simulink model "ForcedPendulum"  (R2023a)
settings: Solver=VariableStepAuto  StartTime=0.0  StopTime=10.0  RelTol=1e-3
model workspace (MAT data in the model file):
  g = 9.8
  l = 0.5
settings Model: Creator=MY PC  LastModifiedBy=MY PC

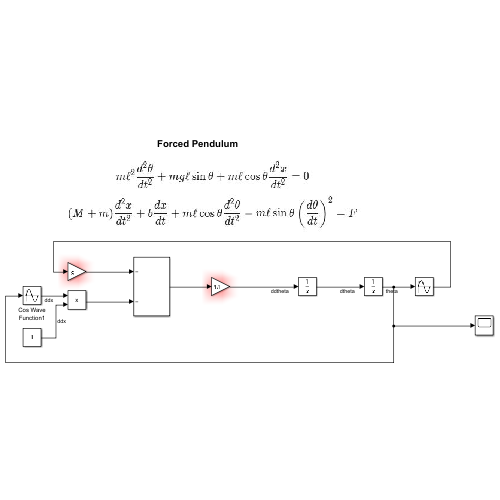
[thumbnail: Simulink's stored preview of the top-level diagram]
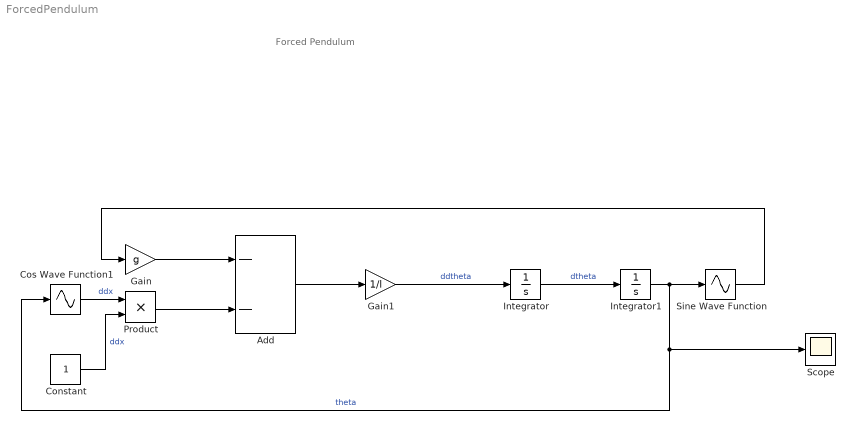
== system ForcedPendulum ==
  note: Forced Pendulum
  Add : Sum  Inputs=--
  Constant : Constant
  Cos Wave Function1 : Sin  TimeSource=Use external signal  Phase=pi/2  SampleTime=0
  Gain : Gain  Gain=g
  Gain1 : Gain  Gain=1/l
  Integrator : Integrator
  Integrator1 : Integrator  InitialCondition=0.9*pi
  Product : Product
  Scope : Scope
  Sine Wave Function : Sin  TimeSource=Use external signal  SampleTime=0
  wires:
  Sine Wave Function/1 -> Gain/1
  Product/1 -> Add/2
  Constant/1 -> Product/2  "ddx"
  Gain1/1 -> Integrator/1  "ddtheta"
  Add/1 -> Gain1/1
  Integrator1/1 -> Cos Wave Function1/1, Scope/1, Sine Wave Function/1  "theta"
  Gain/1 -> Add/1
  Integrator/1 -> Integrator1/1  "dtheta"
  Cos Wave Function1/1 -> Product/1  "ddx"
